simulink model "robot_simple_balancing"  (R2019b)
settings: Solver=ode4  StartTime=0.0  StopTime=10  FixedStep=Ts  RelTol=1e-3
InitFcn:
  | robot_balancing_init
values from neighbouring files (symbols this model uses):
  amplitude_x = 15*pi/180    (= 0.261799387799)    [husky_balancing_init.m]    (also in robot_balancing_init.m = 0.174532925199)
  amplitude_y = 10*pi/180    (= 0.174532925199)    [husky_balancing_init.m]    (also in robot_balancing_init.m)
  amplitude_z = 45*pi/180    (= 0.785398163397)    [husky_balancing_init.m]    (also in robot_balancing_init.m = 0.872664625997)
  desired_q = zeros(1,16)    [robot_balancing_init.m]
  f_x = 4*pi    (= 12.5663706144)    [husky_balancing_init.m]    (also in robot_balancing_init.m = 5)
  f_y = 2*pi    (= 6.28318530718)    [husky_balancing_init.m]    (also in robot_balancing_init.m = 5)
  f_z = 2*pi    (= 6.28318530718)    [husky_balancing_init.m]    (also in robot_balancing_init.m = 1)
  gain = 1    [husky_balancing_init.m]    (also in robot_balancing_init.m = 6)
  p_show = [0.3;-0.2;0]    [robot_balancing_init.m]
undefined symbols (not defined in the file or in its folder): desired_leg, dof, X, Y, Z
libraries: nesl_utility x96, sm_lib x93, Contact_Forces_Lib x4
(part 7 of 7)

== system robot_simple_balancing/Target Motion/leg_top_vis1/Subsystem3 ==
  In1 : Inport
  Cartesian Joint1 : sm_lib/Joints/Cartesian Joint  JointMode=Normal  SenseConstraintForce=off  SenseConstraintForceX=off  SenseConstraintForceY=off  SenseConstraintForceZ=off  SenseConstraintTorque=off  SenseConstraintTorqueX=off  SenseConstraintTorqueY=off  SenseConstraintTorqueZ=off  SenseTotalForce=off  SenseTotalForceX=off  SenseTotalForceY=off  SenseTotalForceZ=off  SenseTotalTorque=off  SenseTotalTorqueX=off  SenseTotalTorqueY=off  SenseTotalTorqueZ=off  CompositeWrenchDir=FollowerOnBase  CompositeWrenchFrame=BaseFrame  PxEquilibriumPosition=0  PxEquilibriumPositionUnits=m  PxSpringStiffness=0  PxSpringStiffnessUnits=N/m  PxDampingCoefficient=0  PxDampingCoefficientUnits=N/(m/s)  PxTorqueActuationMode=ComputedTorque  PxMotionActuationMode=InputMotion  PxSensePosition=off  PxSenseVelocity=off  PxSenseAcceleration=off  PxSenseTorqueForce=off  PxSenseLowerLimitTorqueForce=off  PxSenseUpperLimitTorqueForce=off  PxLowerLimitSpecify=off  PxLowerLimitBound=-1  PxLowerLimitBoundUnits=m  PxLowerLimitStiffness=1e6  PxLowerLimitStiffnessUnits=N/m  PxLowerLimitDamping=1e3  PxLowerLimitDampingUnits=N/(m/s)  PxLowerLimitTransitionRegionWidth=1e-4  PxLowerLimitTransitionRegionWidthUnits=m  PxUpperLimitSpecify=off  PxUpperLimitBound=1  PxUpperLimitBoundUnits=m  PxUpperLimitStiffness=1e6  PxUpperLimitStiffnessUnits=N/m  PxUpperLimitDamping=1e3  PxUpperLimitDampingUnits=N/(m/s)  PxUpperLimitTransitionRegionWidth=1e-4  PxUpperLimitTransitionRegionWidthUnits=m  PxPositionTargetSpecify=off  PxPositionTargetPriority=High  PxPositionTargetValue=0  PxPositionTargetValueUnits=m  PxVelocityTargetSpecify=off  PxVelocityTargetPriority=High  PxVelocityTargetValue=0  PxVelocityTargetValueUnits=m/s  PyEquilibriumPosition=0  PyEquilibriumPositionUnits=m  PySpringStiffness=0  PySpringStiffnessUnits=N/m  PyDampingCoefficient=0  PyDampingCoefficientUnits=N/(m/s)  PyTorqueActuationMode=ComputedTorque  PyMotionActuationMode=InputMotion  PySensePosition=off  PySenseVelocity=off  PySenseAcceleration=off  PySenseTorqueForce=off  PySenseLowerLimitTorqueForce=off  PySenseUpperLimitTorqueForce=off  PyLowerLimitSpecify=off  PyLowerLimitBound=-1  PyLowerLimitBoundUnits=m  PyLowerLimitStiffness=1e6  PyLowerLimitStiffnessUnits=N/m  PyLowerLimitDamping=1e3  PyLowerLimitDampingUnits=N/(m/s)  PyLowerLimitTransitionRegionWidth=1e-4  PyLowerLimitTransitionRegionWidthUnits=m  PyUpperLimitSpecify=off  PyUpperLimitBound=1  PyUpperLimitBoundUnits=m  PyUpperLimitStiffness=1e6  PyUpperLimitStiffnessUnits=N/m  PyUpperLimitDamping=1e3  PyUpperLimitDampingUnits=N/(m/s)  PyUpperLimitTransitionRegionWidth=1e-4  PyUpperLimitTransitionRegionWidthUnits=m  PyPositionTargetSpecify=off  PyPositionTargetPriority=High  PyPositionTargetValue=0  PyPositionTargetValueUnits=m  PyVelocityTargetSpecify=off  PyVelocityTargetPriority=High  PyVelocityTargetValue=0  PyVelocityTargetValueUnits=m/s  PzEquilibriumPosition=0  PzEquilibriumPositionUnits=m  PzSpringStiffness=0  PzSpringStiffnessUnits=N/m  PzDampingCoefficient=0  PzDampingCoefficientUnits=N/(m/s)  PzTorqueActuationMode=ComputedTorque  PzMotionActuationMode=InputMotion  PzSensePosition=off  PzSenseVelocity=off  PzSenseAcceleration=off  PzSenseTorqueForce=off  PzSenseLowerLimitTorqueForce=off  PzSenseUpperLimitTorqueForce=off  PzLowerLimitSpecify=off  PzLowerLimitBound=-1  PzLowerLimitBoundUnits=m  PzLowerLimitStiffness=1e6  PzLowerLimitStiffnessUnits=N/m  PzLowerLimitDamping=1e3  PzLowerLimitDampingUnits=N/(m/s)  PzLowerLimitTransitionRegionWidth=1e-4  PzLowerLimitTransitionRegionWidthUnits=m  PzUpperLimitSpecify=off  PzUpperLimitBound=1  PzUpperLimitBoundUnits=m  PzUpperLimitStiffness=1e6  PzUpperLimitStiffnessUnits=N/m  PzUpperLimitDamping=1e3  PzUpperLimitDampingUnits=N/(m/s)  PzUpperLimitTransitionRegionWidth=1e-4  PzUpperLimitTransitionRegionWidthUnits=m  PzPositionTargetSpecify=off  PzPositionTargetPriority=High  PzPositionTargetValue=0  PzPositionTargetValueUnits=m  PzVelocityTargetSpecify=off  PzVelocityTargetPriority=High  PzVelocityTargetValue=0  PzVelocityTargetValueUnits=m/s
  Demux : Demux  Outputs=3
  SPConv6 : nesl_utility/Simulink-PS Converter  PhysicalDomain=network_engine_domain  SubClassName=ps_input  LeftPortType=input  RightPortType=output  PseudoPeriodic=off  Frequencies=[]  NoiseDistribution=none  NoiseParameters=[]  Unit=m  AffineConversion=off  FilteringAndDerivatives=filter  SimscapeFilterOrder=2  InputFilterTimeConstant=0.001  UdotUserProvided=1
  SPConv7 : nesl_utility/Simulink-PS Converter  PhysicalDomain=network_engine_domain  SubClassName=ps_input  LeftPortType=input  RightPortType=output  PseudoPeriodic=off  Frequencies=[]  NoiseDistribution=none  NoiseParameters=[]  Unit=m  AffineConversion=off  FilteringAndDerivatives=filter  SimscapeFilterOrder=2  InputFilterTimeConstant=0.001  UdotUserProvided=1
  SPConv8 : nesl_utility/Simulink-PS Converter  PhysicalDomain=network_engine_domain  SubClassName=ps_input  LeftPortType=input  RightPortType=output  PseudoPeriodic=off  Frequencies=[]  NoiseDistribution=none  NoiseParameters=[]  Unit=m  AffineConversion=off  FilteringAndDerivatives=filter  SimscapeFilterOrder=2  InputFilterTimeConstant=0.001  UdotUserProvided=1
  Spherical Solid3 : sm_lib/Body Elements/Spherical Solid  GraphicAmbientColor=[0.15 0.15 0.15 1.0]  BasedOnType=Mass  CenterOfMass=[0 0 0]  CenterOfMassUnits=m  GraphicDiffuseColor=[1.0 0.0 0.2]  Density=1000  DensityUnits=kg/m^3  DoExposeReferenceFrame=on  GraphicEmissiveColor=[0.0 0.0 0.0 1.0]  ExportEntireGeometry=off  SerializedExposedGeometries=<ExposedGeometries/>  SerializedFrames=<Frames/>  MarkerShape=Sphere  MarkerSize=10  GraphicType=FromGeometry  InertiaType=CalculateFromGeometry  Mass=0.00001  MassUnits=kg  MomentsOfInertia=[1 1 1]  MomentsOfInertiaUnits=kg*m^2  GraphicOpacity=1.0  ProductsOfInertia=[0 0 0]  ProductsOfInertiaUnits=kg*m^2  GraphicShininess=75  GraphicSpecularColor=[0.5 0.5 0.5 1.0]  SphereRadius=4  SphereRadiusUnits=cm  GraphicVisPropType=SimpleVisualProperties
      settings: SourceProductName=Simscape Multibody
  Connection Port : PMIOPort  Tag=PMCPort  Side=Left
  wires:
  In1/1 -> Demux/1
  Demux/1 -> SPConv6/1
  Demux/2 -> SPConv7/1
  Demux/3 -> SPConv8/1
  connections:
  Cartesian Joint1/RConn1 -- Spherical Solid3/RConn1
  SPConv7/RConn1 -- Cartesian Joint1/LConn3
  SPConv8/RConn1 -- Cartesian Joint1/LConn4
  SPConv6/RConn1 -- Cartesian Joint1/LConn2
  Connection Port/RConn1 -- Cartesian Joint1/LConn1

== system robot_simple_balancing/Target Motion/leg_top_vis1/Subsystem4 ==
  In1 : Inport
  Cartesian Joint1 : sm_lib/Joints/Cartesian Joint  JointMode=Normal  SenseConstraintForce=off  SenseConstraintForceX=off  SenseConstraintForceY=off  SenseConstraintForceZ=off  SenseConstraintTorque=off  SenseConstraintTorqueX=off  SenseConstraintTorqueY=off  SenseConstraintTorqueZ=off  SenseTotalForce=off  SenseTotalForceX=off  SenseTotalForceY=off  SenseTotalForceZ=off  SenseTotalTorque=off  SenseTotalTorqueX=off  SenseTotalTorqueY=off  SenseTotalTorqueZ=off  CompositeWrenchDir=FollowerOnBase  CompositeWrenchFrame=BaseFrame  PxEquilibriumPosition=0  PxEquilibriumPositionUnits=m  PxSpringStiffness=0  PxSpringStiffnessUnits=N/m  PxDampingCoefficient=0  PxDampingCoefficientUnits=N/(m/s)  PxTorqueActuationMode=ComputedTorque  PxMotionActuationMode=InputMotion  PxSensePosition=off  PxSenseVelocity=off  PxSenseAcceleration=off  PxSenseTorqueForce=off  PxSenseLowerLimitTorqueForce=off  PxSenseUpperLimitTorqueForce=off  PxLowerLimitSpecify=off  PxLowerLimitBound=-1  PxLowerLimitBoundUnits=m  PxLowerLimitStiffness=1e6  PxLowerLimitStiffnessUnits=N/m  PxLowerLimitDamping=1e3  PxLowerLimitDampingUnits=N/(m/s)  PxLowerLimitTransitionRegionWidth=1e-4  PxLowerLimitTransitionRegionWidthUnits=m  PxUpperLimitSpecify=off  PxUpperLimitBound=1  PxUpperLimitBoundUnits=m  PxUpperLimitStiffness=1e6  PxUpperLimitStiffnessUnits=N/m  PxUpperLimitDamping=1e3  PxUpperLimitDampingUnits=N/(m/s)  PxUpperLimitTransitionRegionWidth=1e-4  PxUpperLimitTransitionRegionWidthUnits=m  PxPositionTargetSpecify=off  PxPositionTargetPriority=High  PxPositionTargetValue=0  PxPositionTargetValueUnits=m  PxVelocityTargetSpecify=off  PxVelocityTargetPriority=High  PxVelocityTargetValue=0  PxVelocityTargetValueUnits=m/s  PyEquilibriumPosition=0  PyEquilibriumPositionUnits=m  PySpringStiffness=0  PySpringStiffnessUnits=N/m  PyDampingCoefficient=0  PyDampingCoefficientUnits=N/(m/s)  PyTorqueActuationMode=ComputedTorque  PyMotionActuationMode=InputMotion  PySensePosition=off  PySenseVelocity=off  PySenseAcceleration=off  PySenseTorqueForce=off  PySenseLowerLimitTorqueForce=off  PySenseUpperLimitTorqueForce=off  PyLowerLimitSpecify=off  PyLowerLimitBound=-1  PyLowerLimitBoundUnits=m  PyLowerLimitStiffness=1e6  PyLowerLimitStiffnessUnits=N/m  PyLowerLimitDamping=1e3  PyLowerLimitDampingUnits=N/(m/s)  PyLowerLimitTransitionRegionWidth=1e-4  PyLowerLimitTransitionRegionWidthUnits=m  PyUpperLimitSpecify=off  PyUpperLimitBound=1  PyUpperLimitBoundUnits=m  PyUpperLimitStiffness=1e6  PyUpperLimitStiffnessUnits=N/m  PyUpperLimitDamping=1e3  PyUpperLimitDampingUnits=N/(m/s)  PyUpperLimitTransitionRegionWidth=1e-4  PyUpperLimitTransitionRegionWidthUnits=m  PyPositionTargetSpecify=off  PyPositionTargetPriority=High  PyPositionTargetValue=0  PyPositionTargetValueUnits=m  PyVelocityTargetSpecify=off  PyVelocityTargetPriority=High  PyVelocityTargetValue=0  PyVelocityTargetValueUnits=m/s  PzEquilibriumPosition=0  PzEquilibriumPositionUnits=m  PzSpringStiffness=0  PzSpringStiffnessUnits=N/m  PzDampingCoefficient=0  PzDampingCoefficientUnits=N/(m/s)  PzTorqueActuationMode=ComputedTorque  PzMotionActuationMode=InputMotion  PzSensePosition=off  PzSenseVelocity=off  PzSenseAcceleration=off  PzSenseTorqueForce=off  PzSenseLowerLimitTorqueForce=off  PzSenseUpperLimitTorqueForce=off  PzLowerLimitSpecify=off  PzLowerLimitBound=-1  PzLowerLimitBoundUnits=m  PzLowerLimitStiffness=1e6  PzLowerLimitStiffnessUnits=N/m  PzLowerLimitDamping=1e3  PzLowerLimitDampingUnits=N/(m/s)  PzLowerLimitTransitionRegionWidth=1e-4  PzLowerLimitTransitionRegionWidthUnits=m  PzUpperLimitSpecify=off  PzUpperLimitBound=1  PzUpperLimitBoundUnits=m  PzUpperLimitStiffness=1e6  PzUpperLimitStiffnessUnits=N/m  PzUpperLimitDamping=1e3  PzUpperLimitDampingUnits=N/(m/s)  PzUpperLimitTransitionRegionWidth=1e-4  PzUpperLimitTransitionRegionWidthUnits=m  PzPositionTargetSpecify=off  PzPositionTargetPriority=High  PzPositionTargetValue=0  PzPositionTargetValueUnits=m  PzVelocityTargetSpecify=off  PzVelocityTargetPriority=High  PzVelocityTargetValue=0  PzVelocityTargetValueUnits=m/s
  Demux : Demux  Outputs=3
  SPConv6 : nesl_utility/Simulink-PS Converter  PhysicalDomain=network_engine_domain  SubClassName=ps_input  LeftPortType=input  RightPortType=output  PseudoPeriodic=off  Frequencies=[]  NoiseDistribution=none  NoiseParameters=[]  Unit=m  AffineConversion=off  FilteringAndDerivatives=filter  SimscapeFilterOrder=2  InputFilterTimeConstant=0.001  UdotUserProvided=1
  SPConv7 : nesl_utility/Simulink-PS Converter  PhysicalDomain=network_engine_domain  SubClassName=ps_input  LeftPortType=input  RightPortType=output  PseudoPeriodic=off  Frequencies=[]  NoiseDistribution=none  NoiseParameters=[]  Unit=m  AffineConversion=off  FilteringAndDerivatives=filter  SimscapeFilterOrder=2  InputFilterTimeConstant=0.001  UdotUserProvided=1
  SPConv8 : nesl_utility/Simulink-PS Converter  PhysicalDomain=network_engine_domain  SubClassName=ps_input  LeftPortType=input  RightPortType=output  PseudoPeriodic=off  Frequencies=[]  NoiseDistribution=none  NoiseParameters=[]  Unit=m  AffineConversion=off  FilteringAndDerivatives=filter  SimscapeFilterOrder=2  InputFilterTimeConstant=0.001  UdotUserProvided=1
  Spherical Solid3 : sm_lib/Body Elements/Spherical Solid  GraphicAmbientColor=[0.15 0.15 0.15 1.0]  BasedOnType=Mass  CenterOfMass=[0 0 0]  CenterOfMassUnits=m  GraphicDiffuseColor=[1.0 0.0 0.2]  Density=1000  DensityUnits=kg/m^3  DoExposeReferenceFrame=on  GraphicEmissiveColor=[0.0 0.0 0.0 1.0]  ExportEntireGeometry=off  SerializedExposedGeometries=<ExposedGeometries/>  SerializedFrames=<Frames/>  MarkerShape=Sphere  MarkerSize=10  GraphicType=FromGeometry  InertiaType=CalculateFromGeometry  Mass=0.00001  MassUnits=kg  MomentsOfInertia=[1 1 1]  MomentsOfInertiaUnits=kg*m^2  GraphicOpacity=1.0  ProductsOfInertia=[0 0 0]  ProductsOfInertiaUnits=kg*m^2  GraphicShininess=75  GraphicSpecularColor=[0.5 0.5 0.5 1.0]  SphereRadius=4  SphereRadiusUnits=cm  GraphicVisPropType=SimpleVisualProperties
      settings: SourceProductName=Simscape Multibody
  Connection Port : PMIOPort  Tag=PMCPort  Side=Left
  wires:
  In1/1 -> Demux/1
  Demux/1 -> SPConv6/1
  Demux/2 -> SPConv7/1
  Demux/3 -> SPConv8/1
  connections:
  Cartesian Joint1/RConn1 -- Spherical Solid3/RConn1
  SPConv7/RConn1 -- Cartesian Joint1/LConn3
  SPConv8/RConn1 -- Cartesian Joint1/LConn4
  SPConv6/RConn1 -- Cartesian Joint1/LConn2
  Connection Port/RConn1 -- Cartesian Joint1/LConn1

== matlab function robot_simple_balancing/Controller ==
  data: R input; enable input; d_leg output; desired_q parameter; gain parameter
function d_leg  = fcn(R,enable, desired_q,gain)
%     R=rotm_x_h(q(1))*rotm_y_h(q(2))*rotm_z_h(q(3));
         alpha=rotm2eul(R,'XYZ')
         R=eul2rotm(alpha.*gain,'XYZ');
%         alpha=alpha.*[-1,1,1];
%         R_converted=eul2rotm(alpha,'XYZ');
        T_FR=[eye(3,3),[0.3;-0.2;0];0,0,0,1];
        T_FL=[eye(3,3),[0.3;0.2;0];0,0,0,1];
        T_BR=[eye(3,3),[-0.3;-0.2;0];0,0,0,1];
        T_BL=[eye(3,3),[-0.3;0.2;0];0,0,0,1];
        
        R_FR=[eul2rotm(desired_q(1:3),'XYZ'),[0;0;0];0,0,0,1];
        R_FL=[eul2rotm(desired_q(5:7),'XYZ'),[0;0;0];0,0,0,1];
        R_BR=[eul2rotm(desired_q(9:11),'XYZ'),[0;0;0];0,0,0,1];
        R_BL=[eul2rotm(desired_q(13:15),'XYZ'),[0;0;0];0,0,0,1];
        
        p_FR_temp=T_FR*R_FR*[0;0;desired_q(4);1];
        p_FL_temp=T_FL*R_FL*[0;0;desired_q(8);1];
        p_BR_temp=T_BR*R_BR*[0;0;desired_q(12);1];
        p_BL_temp=T_BL*R_BL*[0;0;desired_q(16);1];
        
        p_FR_e=p_FR_temp(1:3)-[0;0;p_FR_temp(3)];
        p_FL_e=p_FL_temp(1:3)-[0;0;p_FL_temp(3)];
        p_BR_e=p_BR_temp(1:3)-[0;0;p_BR_temp(3)];
        p_BL_e=p_BL_temp(1:3)-[0;0;p_BL_temp(3)];
        
        p_e=[p_FR_e,p_FL_e,p_BR_e,p_BL_e]
        
        p_FR_t=[0.3;-0.2;-p_FR_temp(3)];
        p_FL_t=[0.3;0.2;-p_FL_temp(3)];
        p_BR_t=[-0.3;-0.2;-p_BR_temp(3)];
        p_BL_t=[-0.3;0.2;-p_BL_temp(3)];
        
        p_t=[p_FR_t,p_FL_t,p_BR_t,p_BL_t]
        d_leg=zeros(1,16);
    if enable
        p_e_new=inv(R')*p_e;
        p_t_new=inv(R)*p_t;
%         d_leg=zeros(1,16);
%         for i=1:4
        for i=1:4
            p1=p_t(:,i);
            p2=p_e(:,i);
            p1_new=p_t_new(:,i);
            p2_new=p_e_new(:,i);
            old_leg_length=norm(p2-p1);
            new_leg_length=norm(p2_new-p1);
%             u=p1-p2;
            v=p2_new-p1;
%             error=u-v
            quat=vec2quat([0;0;desired_q(4*i)],v);
            euler_angle=quat2eul(quat,'XYZ');
            d_leg(4*i-3:4*i-1)=euler_angle;
            d_leg(4*i)=-(new_leg_length-old_leg_length)+desired_q(4*i);
        end
    else
        p_t_new=p_t;
        p_e_new=p_e;
        d_leg=desired_q;
    end
end

function rotm=rotm_x_h(theta)
    rotm=[1,0,0;0,cos(theta),sin(theta);0,-sin(theta),cos(theta)];
end

function rotm=rotm_y_h(theta)
    rotm=[cos(theta),0,sin(theta);0,1,0;-sin(theta),0,cos(theta)];
end

function rotm=rotm_z_h(theta)
    rotm=[cos(theta),-sin(theta),0;sin(theta),cos(theta),0;0,0,1];
end

function q=vec2quat(p1,p2)
    p1=p1./norm(p1);
    p2=p2./norm(p2);
    if p1==p2
        q=[1,0,0,0];
    else
    u = cross(p1,p2)/norm(cross(p1,p2));
    alpha = acos(dot(p1,p2)/(norm(p1)*norm(p2)));
    q = [cos(alpha/2), sin(alpha/2)*u(1), sin(alpha/2)*u(2), sin(alpha/2)*u(3)];
    end
end

== matlab function robot_simple_balancing/Tracking Test/MATLAB Function1 ==
  data: q_out output; q input; x output
function [q_out,x] = fcn(q)
    T_FR=[eye(3,3),[0.3;-0.2;0];0,0,0,1];
    R=[eul2rotm(q(1:3)','XYZ'),[0;0;0];0,0,0,1];
    x_temp=T_FR*R*[0;0;q(4);1];
	x=x_temp(1:3);
    quat=vec2quat([0;0;q(4)],x-[0.3;-0.2;0]);
    q_out=[quat2eul(quat,'XYZ'),q(4)];
end
    
    
function q=vec2quat(p1,p2)
if p1==p2
        q=[1,0,0,0];
    else
    u = cross(p1,p2)/norm(cross(p1,p2));
    alpha = acos(dot(p1,p2)/(norm(p1)*norm(p2)));
    q = [cos(alpha/2), sin(alpha/2)*u(1), sin(alpha/2)*u(2), sin(alpha/2)*u(3)]
end
end
